simulink model "untitled"  (R2021b)
settings: Solver=VariableStepAuto  StartTime=0.0  StopTime=10.0  RelTol=1e-3
settings Model: Creator=danli  LastModifiedBy=danli

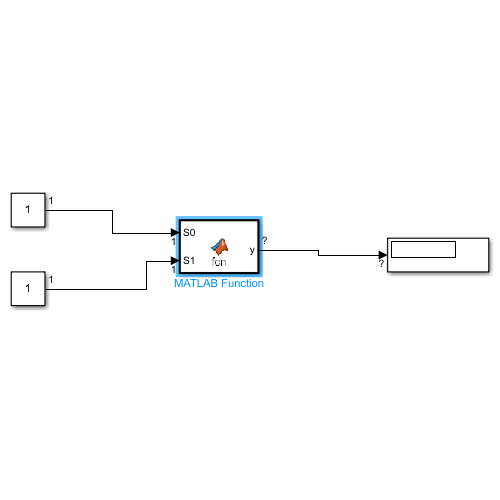
[thumbnail: Simulink's stored preview of the top-level diagram]
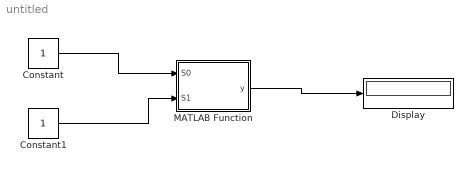
== system untitled ==
  Constant : Constant
  Constant1 : Constant
  Display : Display
  MATLAB Function : MATLAB Function  TreatAsAtomicUnit=on
  wires:
  Constant/1 -> MATLAB Function/1(S0)
  Constant1/1 -> MATLAB Function/2(S1)
  MATLAB Function/1(y) -> Display/1

== matlab function untitled/MATLAB Function ==
  data: S0 input; y output; S1 input
function y = fcn(S0,S1)

y = -(4071944862313895276541*S0*S1^2)/140737488355328000000;
